simulink model "agent_model"  (R2020b)
settings: Solver=VariableStepAuto  StartTime=0.0  StopTime=10.0  RelTol=1e-3
values from neighbouring files (symbols this model uses):
  A_plant = [0 1; 880.87 0]    [alternative_model.m]    (also in alternative_model_script.m; observer_convergence.m; p1.m; stable_template.m)
  B_plant = [0; -9.9453]    [alternative_model.m]    (also in alternative_model_script.m; observer_convergence.m; p1.m; stable_template.m)
  c = 10/den    [alternative_model.m]    (also in alternative_model_script.m; p1.m = 100/den; stable_template.m; template.m)
  C_plant = [708.27 0]    [alternative_model.m]    (also in alternative_model_script.m; observer_convergence.m; p1.m; stable_template.m)
  K = B'/R*P    [alternative_model.m]    (also in alternative_model_script.m; free_response.m = sym('K', [2,2]); p1.m; stable_template.m)
  K_plant = acker(A_plant, B_plant, poles)    [alternative_model.m]    (also in alternative_model_script.m; p1.m; stable_template.m; template.m)
  output_state = 1    [v1.m]
  x0_agent = [0.1 2]    [alternative_model.m]    (also in alternative_model_script.m; p1.m = [0 0]; stable_template.m = [0 0]; template.m = [0 0])
libraries: simulink x1
settings Model: Creator=salvo  LastModifiedBy=salvo
settings ModelReferenceCC: ModelReferenceMinAlgLoopOccurrences=on

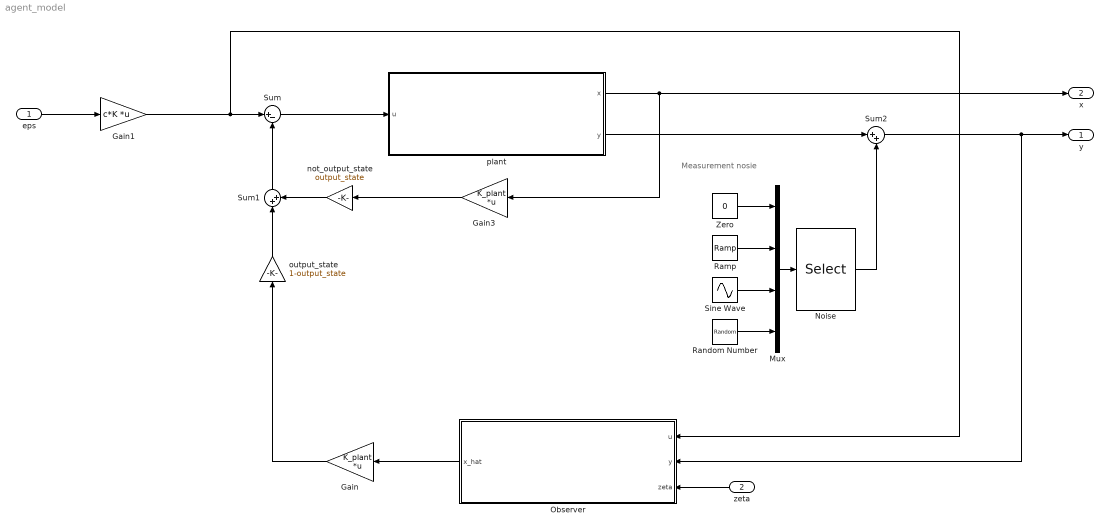
== system agent_model ==
  note: Measurement nosie
  eps : Inport  PortDimensions=2
  zeta : Inport  Port=2
  Gain : Gain  Gain=K_plant  Multiplication=Matrix(K*u)
  Gain1 : Gain  Gain=c*K  Multiplication=Matrix(K*u)
  Gain3 : Gain  Gain=K_plant  Multiplication=Matrix(K*u)
  Mux : Mux
  Noise : Selector  InputPortWidth=4  IndexOptions=Index vector (dialog)  Indices=measurement_noise_type  OutputSizes=1
  Observer : Subsystem
  Ramp : simulink/Sources/Ramp  slope=1  start=0  InitialOutput=0
  Random Number : RandomNumber  SampleTime=0.1
  Sine Wave : Sin  SampleTime=0
  Sum : Sum  Inputs=|+-
  Sum1 : Sum  Inputs=|++
  Sum2 : Sum  Inputs=|++
  Zero : Constant  Value=0  OutDataTypeStr=Inherit: Inherit via back propagation
  not_output_state : Gain  Gain=output_state
  output_state : Gain  Gain=1-output_state
  plant : Subsystem
  y : Outport
  x : Outport  Port=2
  wires:
  Gain/1 -> output_state/1
  zeta/1 -> Observer/3(zeta)
  eps/1 -> Gain1/1
  Sum/1 -> plant/1(u)
  Observer/1(x_hat) -> Gain/1
  plant/1(x) -> Gain3/1, x/1
  Gain1/1 -> Observer/1(u), Sum/1
  output_state/1 -> Sum1/1
  Sum1/1 -> Sum/2
  not_output_state/1 -> Sum1/2
  Gain3/1 -> not_output_state/1
  plant/2(y) -> Sum2/1
  Zero/1 -> Mux/1
  Noise/1 -> Sum2/2
  Sum2/1 -> Observer/2(y), y/1
  Random Number/1 -> Mux/4
  Ramp/1 -> Mux/2
  Sine Wave/1 -> Mux/3
  Mux/1 -> Noise/1

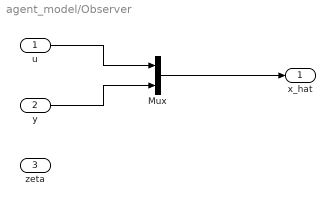
== system agent_model/Observer ==
  u : Inport
  y : Inport  Port=2
  zeta : Inport  Port=3
  Mux : Mux  Inputs=2
  x_hat : Outport
  wires:
  Mux/1 -> x_hat/1
  u/1 -> Mux/1
  y/1 -> Mux/2

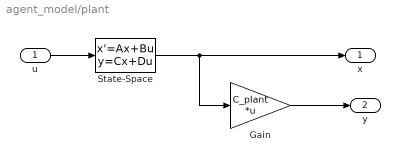
== system agent_model/plant ==
  u : Inport
  Gain : Gain  Gain=C_plant  Multiplication=Matrix(K*u)
  State-Space : StateSpace  A=A_plant  B=B_plant  C=eye(2)  D=[0; 0]  InitialCondition=x0_agent
  x : Outport
  y : Outport  Port=2
  wires:
  u/1 -> State-Space/1
  Gain/1 -> y/1
  State-Space/1 -> x/1, Gain/1
